simulink model "powertrain_modelling_simulation"  (R2023b)
settings: Solver=VariableStepAuto  StartTime=0.0  StopTime=time  RelTol=1e-3
model workspace (MATLAB code in the model file):
  | Rw = 0.254; % radius of vehicle
  | GVM = 330;  % gross vehicle mass(kg)
  | GVW = GVM*9.8; % gross vehicle weight(kg.m/s^2)
  | Crf = 0.015; % coeff of rolling resistance
  | slope_angle = 0; % slope angle in radian
  | Af = 1.1; % frontal Area (m^2)
  | Cd = 0.4; % coeff of drag
  | gear_ratio = 6;
  | trans_eff = 0.9;
  | motor_eff = 0.9;
  | mc_eff = 0.95;
  | Bv = 72; % battery voltage
  | Cv = 3.6; % cell voltage (V)
  | Cc = 31; %cell capacity (Ah)
  | lap_distance = 0.787; % distance of one lap (km)
  | range = 20; % range of vehicle in single charge
  | time = 60; % time required to complete one lap
  | air_density = 1.225 ;
libraries: autolibshared x1

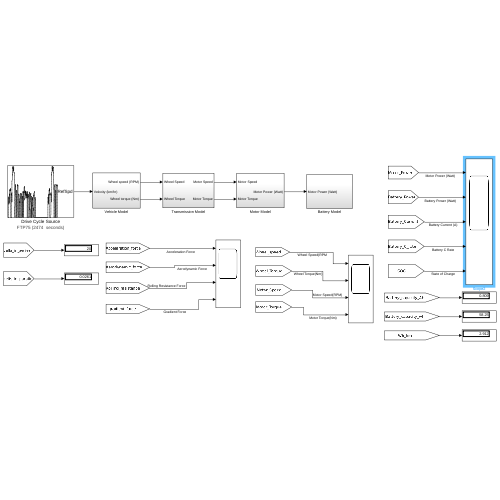
[thumbnail: Simulink's stored preview of the top-level diagram]
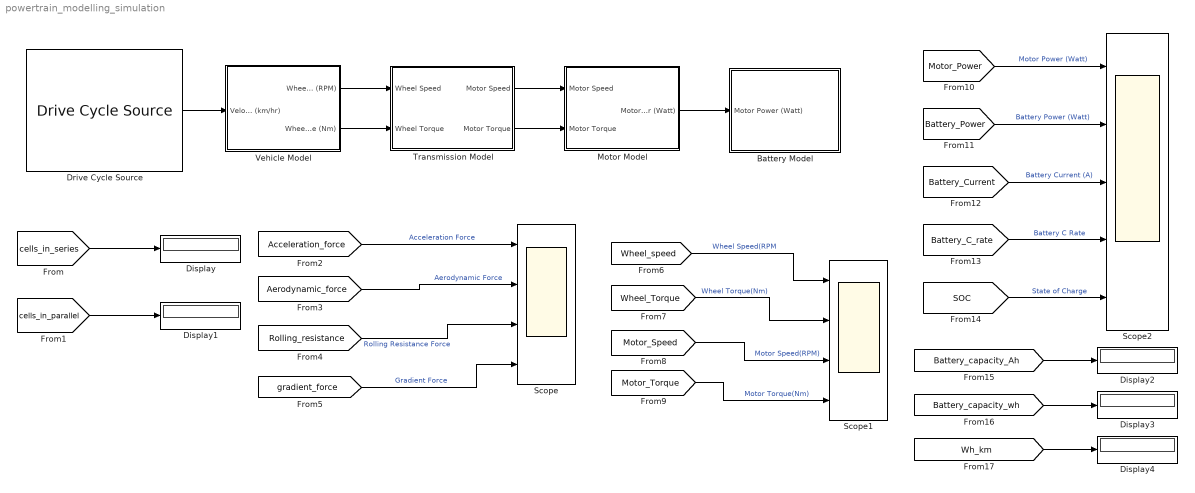
== system powertrain_modelling_simulation ==
  Battery Model : Subsystem
  Display{,1..4} (5 alike) : Display
  Drive Cycle Source : autolibshared/Drive Cycle Source  cycleVar=FTP75  fileVar=cycleFTP75.mat  tfinal="2474  seconds"  cycleRepeat=off  outAccPort=off  outGearPort=off  gearList=No gear data  t_wot1=5  xdot_woto=0  xdot_wot1=30  t_wot2=20  xdot_wot2=0  t_wotend=30  srcUnit=m/s  outUnit=m/s  srcAccUnit=m/s/s  outAccUnit=m/s^2  dt=0  aMode=1  faultOption=off  velBnd=2  velBndUnit=mph  inUnit=m/s  timeBnd=1  failOption=off  stopSim=off  maxFaultCnt=10  maxFaultTime=2  maxTotFaultTime=15  traceOption=off  dtTrace=1  traceWindow=10  lastDCname=FTP75  lastOutUnit=mph  lastDT=0  lastTB=1  lastSB=2  forceCalcBound=off
  Motor Model : Subsystem
  Scope : Scope  NumInputPorts=4
  Scope1 : Scope  NumInputPorts=4
  Scope2 : Scope  NumInputPorts=5
  Transmission Model : Subsystem
  Vehicle Model : Subsystem
  wires:
  Vehicle Model/1(Wheel speed (RPM)) -> Transmission Model/1(Wheel Speed)
  Vehicle Model/2(Wheel torque (Nm)) -> Transmission Model/2(Wheel Torque)
  Transmission Model/1(Motor Speed) -> Motor Model/1(Motor Speed)
  Transmission Model/2(Motor Torque) -> Motor Model/2(Motor Torque)
  Motor Model/1(Motor Power (Watt)) -> Battery Model/1(Motor Power (Watt))
  [cells_in_series] -> Display/1
  [cells_in_parallel] -> Display1/1
  [Acceleration_force] -> Scope/1  "Acceleration Force"
  [Aerodynamic_force] -> Scope/2  "Aerodynamic Force"
  [Rolling_resistance] -> Scope/3  "Rolling Resistance Force"
  [gradient_force] -> Scope/4  "Gradient Force"
  [Wheel_speed] -> Scope1/1  "Wheel Speed(RPM"
  [Wheel_Torque] -> Scope1/2  "Wheel Torque(Nm)"
  [Motor_Speed] -> Scope1/3  "Motor Speed(RPM)"
  [Motor_Torque] -> Scope1/4  "Motor Torque(Nm)"
  [Motor_Power] -> Scope2/1  "Motor Power (Watt)"
  [Battery_Power] -> Scope2/2  "Battery Power (Watt)"
  [Battery_Current] -> Scope2/3  "Battery Current (A)"
  [Battery_C_rate] -> Scope2/4  "Battery C Rate"
  [SOC] -> Scope2/5  "State of Charge"
  [Battery_capacity_Ah] -> Display2/1
  [Wh_km] -> Display4/1
  [Battery_capacity_wh] -> Display3/1
  Drive Cycle Source/1 -> Vehicle Model/1(Velocity (km/hr))

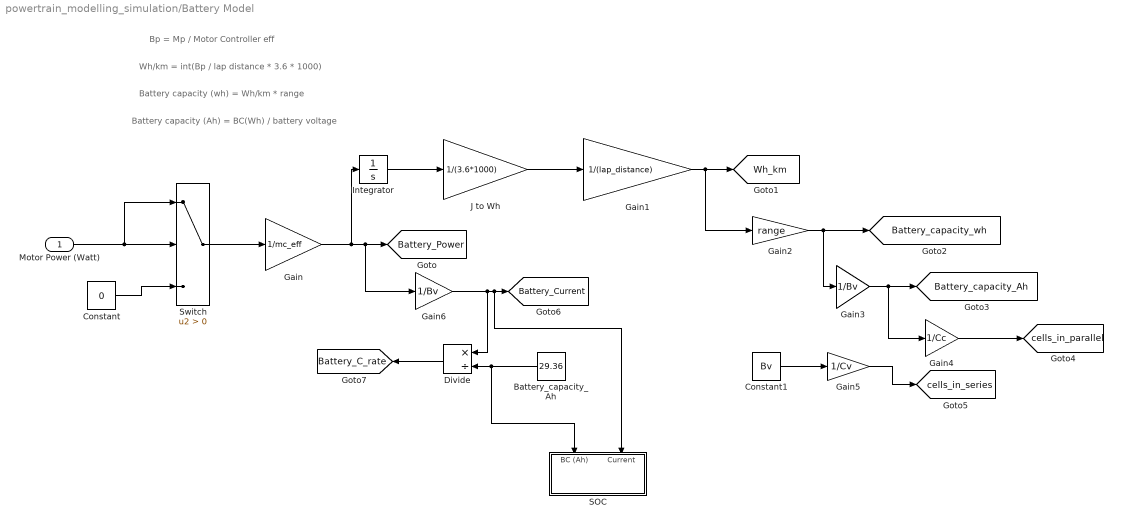
== system powertrain_modelling_simulation/Battery Model ==
  note: Battery capacity (Ah) = BC(Wh) / battery voltage
  note: Battery capacity (wh) = Wh/km * range
  note: Wh/km = int(Bp / lap distance * 3.6 * 1000)
  note: Bp = Mp / Motor Controller eff
  Motor Power (Watt) : Inport
  Battery_capacity_Ah : Constant  Value=29.36
  Constant : Constant  Value=0
  Constant1 : Constant  Value=Bv
  Divide : Product  Inputs=*/
  Gain : Gain  Gain=1/mc_eff
  Gain1 : Gain  Gain=1/(lap_distance)
  Gain2 : Gain  Gain=range
  Gain3 : Gain  Gain=1/Bv
  Gain4 : Gain  Gain=1/Cc
  Gain5 : Gain  Gain=1/Cv
  Gain6 : Gain  Gain=1/Bv
  Integrator : Integrator
  J to Wh : Gain  Gain=1/(3.6*1000)
  SOC : Subsystem
      settings: PortSchema="{\"entries\":[{\"content\":{\"sides\":[{\"content\":{},\"type\":\"ConnectorPlacement.EquallySpacedRectSide\",\"uuid\":\"918ab17c-8ee6-4e28-9e81-e08d3841ca85\"},{\"content\":{\"side\":\"RIGHT\"},\"type\":\"ConnectorPlacement.EquallySpacedRectSide\",\"uuid\":\"b145a5db-ef7a-4d63-afa7-5eae9e4776c8\"},{\"content\":{\"connectorIds\":[\"In1\",\"In2\"],\"side\":\"TOP\"},\"type\":\"ConnectorPlacement.EquallySpacedRectSide\",\"uuid\":\"4de68463-c688-4f6b-891a-3122fd1f387d\"}]},\"type\":\"ConnectorPlacement.EquallySpacedConnector\",\"uuid\":\"a2bcce66-3c9a-4c6d-b49f-8164ae1a2476\"}],\"packageUris\":[\"http://schema.mathworks.com/mf0/Connector/R2020b\"],\"version\":\"1.0\"}"
  Switch : Switch  Criteria=u2 > Threshold  SaturateOnIntegerOverflow=off  InputSameDT=off
  tag scope: Battery_C_rate=global, Battery_Current=global, Battery_Power=global, Battery_capacity_Ah=global, Battery_capacity_wh=global, Wh_km=global, cells_in_parallel=global, cells_in_series=global
  wires:
  Motor Power (Watt)/1 -> Switch/1, Switch/2
  Constant/1 -> Switch/3
  Switch/1 -> Gain/1
  Gain/1 -> Integrator/1, Gain6/1, [Battery_Power]
  Integrator/1 -> J to Wh/1
  J to Wh/1 -> Gain1/1
  Gain1/1 -> Gain2/1, [Wh_km]
  Gain2/1 -> Gain3/1, [Battery_capacity_wh]
  Gain3/1 -> Gain4/1, [Battery_capacity_Ah]
  Gain4/1 -> [cells_in_parallel]
  Constant1/1 -> Gain5/1
  Gain5/1 -> [cells_in_series]
  Gain6/1 -> Divide/1, SOC/2(Current), [Battery_Current]
  Battery_capacity_Ah/1 -> SOC/1(BC (Ah)), Divide/2
  Divide/1 -> [Battery_C_rate]

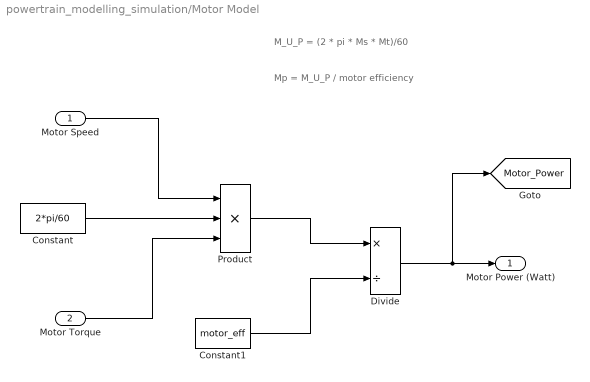
== system powertrain_modelling_simulation/Motor Model ==
  note: Mp = M_U_P / motor efficiency
  note: M_U_P = (2 * pi * Ms * Mt)/60
  Motor Speed : Inport
  Motor Torque : Inport  Port=2
  Constant : Constant  Value=2*pi/60
  Constant1 : Constant  Value=motor_eff
  Divide : Product  Inputs=*/
  Product : Product  Inputs=3
  Motor Power (Watt) : Outport
  tag scope: Motor_Power=global
  wires:
  Motor Speed/1 -> Product/1
  Constant/1 -> Product/2
  Motor Torque/1 -> Product/3
  Product/1 -> Divide/1
  Constant1/1 -> Divide/2
  Divide/1 -> [Motor_Power], Motor Power (Watt)/1

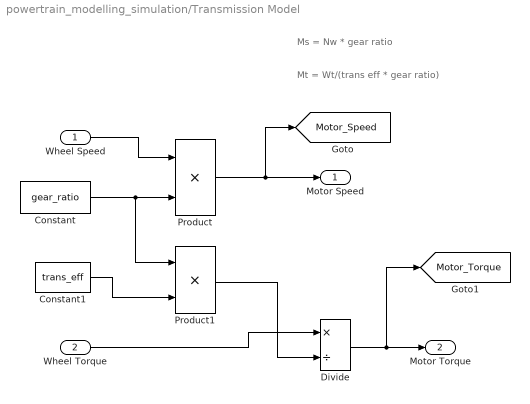
== system powertrain_modelling_simulation/Transmission Model ==
  note: Mt = Wt/(trans eff * gear ratio)
  note: Ms = Nw * gear ratio
  Wheel Speed : Inport
  Wheel Torque : Inport  Port=2
  Constant : Constant  Value=gear_ratio
  Constant1 : Constant  Value=trans_eff
  Divide : Product  Inputs=*/
  Product : Product
  Product1 : Product
  Motor Speed : Outport
  Motor Torque : Outport  Port=2
  tag scope: Motor_Speed=global, Motor_Torque=global
  wires:
  Wheel Speed/1 -> Product/1
  Constant/1 -> Product1/1, Product/2
  Product/1 -> [Motor_Speed], Motor Speed/1
  Constant1/1 -> Product1/2
  Product1/1 -> Divide/2
  Wheel Torque/1 -> Divide/1
  Divide/1 -> [Motor_Torque], Motor Torque/1

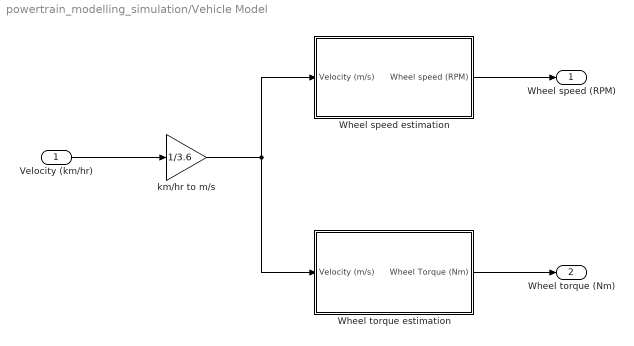
== system powertrain_modelling_simulation/Vehicle Model ==
  Velocity (km/hr) : Inport
  Wheel speed estimation : Subsystem
  Wheel torque estimation : Subsystem
  km/hr to m/s : Gain  Gain=1/3.6
  Wheel speed (RPM) : Outport
  Wheel torque (Nm) : Outport  Port=2
  wires:
  Velocity (km/hr)/1 -> km/hr to m/s/1
  km/hr to m/s/1 -> Wheel speed estimation/1(Velocity (m/s)), Wheel torque estimation/1(Velocity (m/s))
  Wheel speed estimation/1(Wheel speed (RPM)) -> Wheel speed (RPM)/1
  Wheel torque estimation/1(Wheel Torque (Nm)) -> Wheel torque (Nm)/1

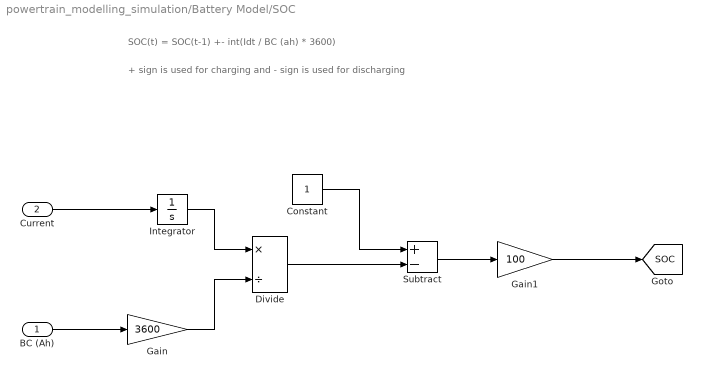
== system powertrain_modelling_simulation/Battery Model/SOC ==
  note: + sign is used for charging and - sign is used for discharging
  note: SOC(t) = SOC(t-1) +- int(Idt / BC (ah) * 3600)
  BC (Ah) : Inport
  Current : Inport  Port=2
  Constant : Constant
  Divide : Product  Inputs=*/
  Gain : Gain  Gain=3600
  Gain1 : Gain  Gain=100
  Integrator : Integrator
  Subtract : Sum  Inputs=+-
  tag scope: SOC=global
  wires:
  BC (Ah)/1 -> Gain/1
  Current/1 -> Integrator/1
  Integrator/1 -> Divide/1
  Gain/1 -> Divide/2
  Constant/1 -> Subtract/1
  Divide/1 -> Subtract/2
  Subtract/1 -> Gain1/1
  Gain1/1 -> [SOC]

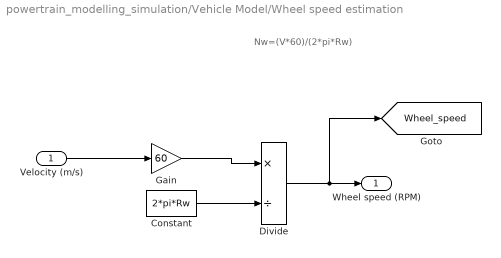
== system powertrain_modelling_simulation/Vehicle Model/Wheel speed estimation ==
  note: Nw=(V*60)/(2*pi*Rw)
  Velocity (m/s) : Inport
  Constant : Constant  Value=2*pi*Rw
  Divide : Product  Inputs=*/
  Gain : Gain  Gain=60
  Wheel speed (RPM) : Outport
  tag scope: Wheel_speed=global
  wires:
  Velocity (m/s)/1 -> Gain/1
  Gain/1 -> Divide/1
  Constant/1 -> Divide/2
  Divide/1 -> [Wheel_speed], Wheel speed (RPM)/1

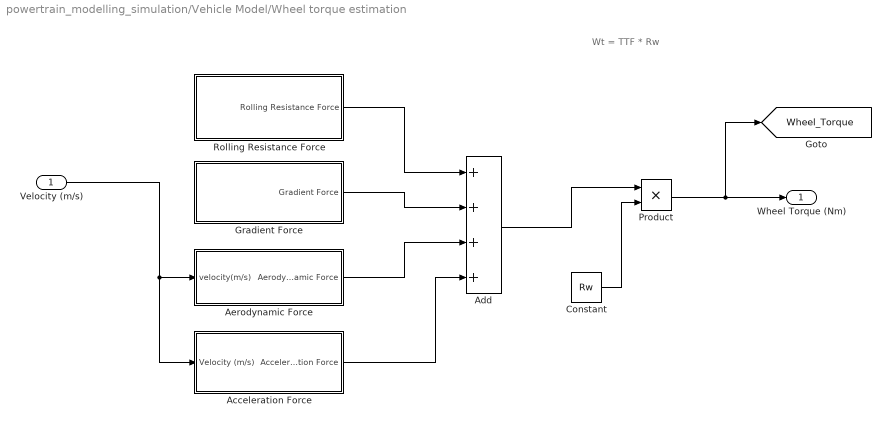
== system powertrain_modelling_simulation/Vehicle Model/Wheel torque estimation ==
  note: Wt = TTF * Rw
  Velocity (m/s) : Inport
  Acceleration Force : Subsystem
  Add : Sum  Inputs=++++
  Aerodynamic Force : Subsystem
  Constant : Constant  Value=Rw
  Gradient Force : Subsystem
  Product : Product
  Rolling Resistance Force : Subsystem
  Wheel Torque (Nm) : Outport
  tag scope: Wheel_Torque=global
  wires:
  Velocity (m/s)/1 -> Acceleration Force/1(Velocity (m/s)), Aerodynamic Force/1(velocity(m/s))
  Rolling Resistance Force/1(Rolling Resistance Force) -> Add/1
  Gradient Force/1(Gradient Force) -> Add/2
  Aerodynamic Force/1(Aerodynamic Force) -> Add/3
  Acceleration Force/1(Acceleration Force) -> Add/4
  Add/1 -> Product/1
  Constant/1 -> Product/2
  Product/1 -> [Wheel_Torque], Wheel Torque (Nm)/1

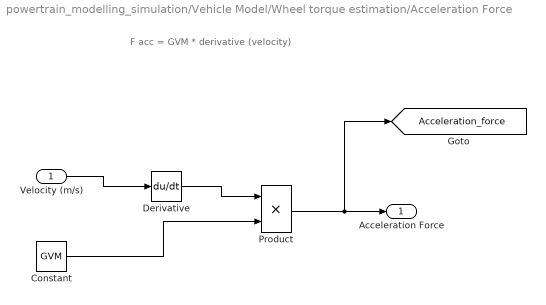
== system powertrain_modelling_simulation/Vehicle Model/Wheel torque estimation/Acceleration Force ==
  note: F acc = GVM * derivative (velocity)
  Velocity (m/s) : Inport
  Constant : Constant  Value=GVM
  Derivative : Derivative
  Product : Product
  Acceleration Force : Outport
  tag scope: Acceleration_force=global
  wires:
  Velocity (m/s)/1 -> Derivative/1
  Derivative/1 -> Product/1
  Constant/1 -> Product/2
  Product/1 -> [Acceleration_force], Acceleration Force/1

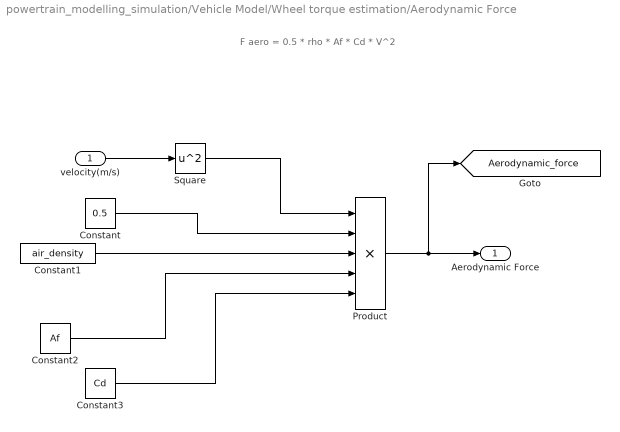
== system powertrain_modelling_simulation/Vehicle Model/Wheel torque estimation/Aerodynamic Force ==
  note: F aero = 0.5 * rho * Af * Cd * V^2
  velocity(m/s) : Inport
  Constant : Constant  Value=0.5
  Constant1 : Constant  Value=air_density
  Constant2 : Constant  Value=Af
  Constant3 : Constant  Value=Cd
  Product : Product  Inputs=5
  Square : Math  Operator=square
  Aerodynamic Force : Outport
  tag scope: Aerodynamic_force=global
  wires:
  velocity(m/s)/1 -> Square/1
  Square/1 -> Product/1
  Constant/1 -> Product/2
  Constant1/1 -> Product/3
  Constant2/1 -> Product/4
  Constant3/1 -> Product/5
  Product/1 -> [Aerodynamic_force], Aerodynamic Force/1

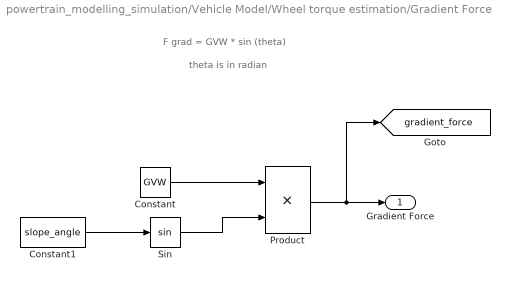
== system powertrain_modelling_simulation/Vehicle Model/Wheel torque estimation/Gradient Force ==
  note: theta is in radian
  note: F grad = GVW * sin (theta)
  Constant : Constant  Value=GVW
  Constant1 : Constant  Value=slope_angle
  Product : Product
  Sin : Trigonometry
  Gradient Force : Outport
  tag scope: gradient_force=global
  wires:
  Constant1/1 -> Sin/1
  Constant/1 -> Product/1
  Sin/1 -> Product/2
  Product/1 -> [gradient_force], Gradient Force/1

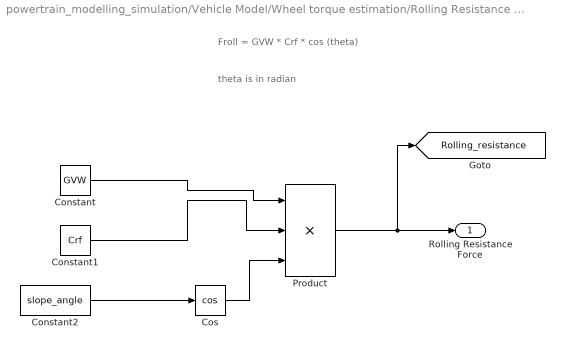
== system powertrain_modelling_simulation/Vehicle Model/Wheel torque estimation/Rolling Resistance Force ==
  note: theta is in radian
  note: Froll = GVW * Crf * cos (theta)
  Constant : Constant  Value=GVW
  Constant1 : Constant  Value=Crf
  Constant2 : Constant  Value=slope_angle
  Cos : Trigonometry  Operator=cos
  Product : Product  Inputs=3
  Rolling Resistance Force : Outport
  tag scope: Rolling_resistance=global
  wires:
  Constant2/1 -> Cos/1
  Constant/1 -> Product/1
  Constant1/1 -> Product/2
  Cos/1 -> Product/3
  Product/1 -> [Rolling_resistance], Rolling Resistance Force/1
